simulink model "Bicopter_Dynamics"  (R2019a)
settings: Solver=ode4  StartTime=0.0  StopTime=5  FixedStep=0.0001  RelTol=1e-3
libraries: simulink x1
settings Model: Creator=crsmyth  LastModifiedBy=crs20

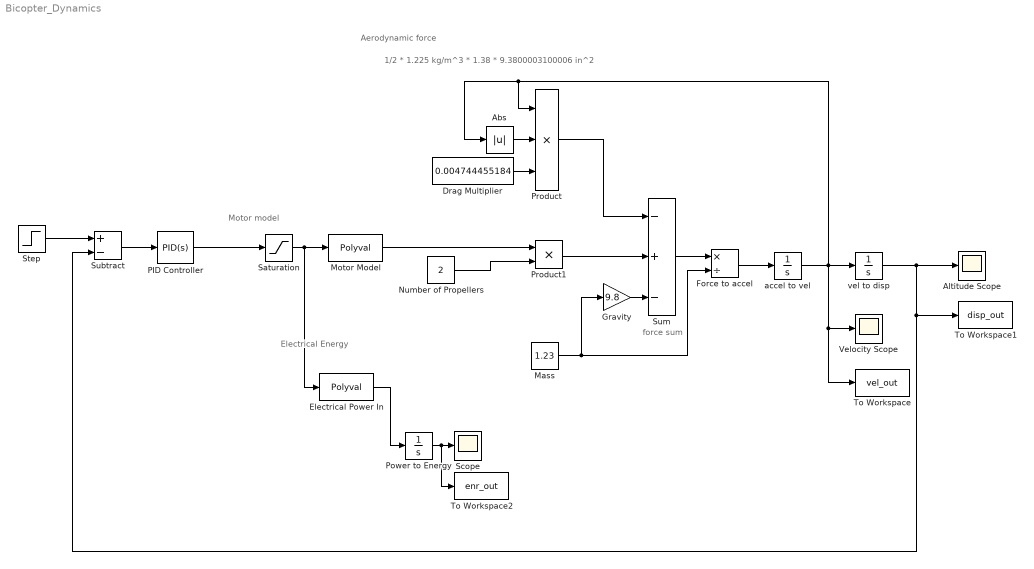
== system Bicopter_Dynamics ==
  note: Electrical Energy
  note: force sum
  note: Motor model
  note: Aerodynamic force
  note: 1/2 * 1.225 kg/m^3 * 1.38 * 9.3800003100006 in^2
  Abs : Abs
  Altitude Scope : Scope
  Drag Multiplier : Constant  Value=0.004744455184
  Electrical Power In : Polyval  Coefs=[2.956191832898671e+02, -6.235353126465623e+02, 3.330393150826374e+02]
  Force to accel : Product  Inputs=*/
  Gravity : Gain  Gain=9.8
  Mass : Constant  Value=1.23
  Motor Model : Polyval  Coefs=[4.843819998761814,-4.792311105872948,-0.068689974553541]
  Number of Propellers : Constant  Value=2
  PID Controller : simulink/Continuous/PID Controller  Controller=PID  Form=Parallel  TimeDomain=Continuous-time  SampleTime=-1  IntegratorMethod=Forward Euler  FilterMethod=Forward Euler  ControllerParametersSource=internal  P=1.5  I=1.3  D=0.3  UseFilter=on  N=10  TunerSelectOption=Transfer Function Based (PID Tuner App)  InitialConditionSource=internal  InitialConditionForIntegrator=0  InitialConditionForFilter=0  DifferentiatorICPrevScaledInput=0  ExternalReset=none  TrackingMode=off  Kt=1  LimitOutput=off  UpperSaturationLimit=inf  LowerSaturationLimit=-inf  LinearizeAsGain=on  AntiWindupMode=none  Kb=1  POutMin=[]  POutMax=[]  IOutMin=[]  IOutMax=[]  DOutMin=[]  DOutMax=[]  NOutMin=[]  NOutMax=[]  SumOutMin=[]  SumOutMax=[]  SaturationOutMin=[]  SaturationOutMax=[]  PParamMin=[]  PParamMax=[]  IParamMin=[]  IParamMax=[]  DParamMin=[]  DParamMax=[]  NParamMin=[]  NParamMax=[]  KbParamMin=[]  KbParamMax=[]  KtParamMin=[]  KtParamMax=[]  KbOutMin=[]  KbOutMax=[]  KtOutMin=[]  KtOutMax=[]  IntegratorOutMin=[]  IntegratorOutMax=[]  FilterOutMin=[]  FilterOutMax=[]  SumI1OutMin=[]  SumI1OutMax=[]  SumI2OutMin=[]  SumI2OutMax=[]  SumI3OutMin=[]  SumI3OutMax=[]  SumI4OutMin=[]  SumI4OutMax=[]  SumDOutMin=[]  SumDOutMax=[]  DifferentiatorOutMin=[]  DifferentiatorOutMax=[]  FilterDiffOutCoefMin=[]  FilterDiffOutCoefMax=[]  ReciprocalOutMin=[]  ReciprocalOutMax=[]  SumDenOutMin=[]  SumDenOutMax=[]  SumNumOutMin=[]  SumNumOutMax=[]  DivideOutMin=[]  DivideOutMax=[]  IntegratorContinuousStateAttributes=''  IntegratorStateMustResolveToSignalObject=off  IntegratorRTWStateStorageClass=Auto  FilterContinuousStateAttributes=''  FilterStateMustResolveToSignalObject=off  FilterRTWStateStorageClass=Auto  ParallelPVariant=InternalParameters  IdealPVariant=Disabled  IVariant=InternalParameters  DVariant=InternalParameters  IntegratorVariant=Continuous  SatVariant=Disabled  AWVariant=Passthrough  PCopyVariant=Disabled  TRVariant=Disabled  FdbkBlocksVariant=Forward  IdealPFdbkVariant=Disabled  SatFdbkVariant=Disabled  DerivativeFilterVariant=ContFilter  NVariant=InternalParameters  NCopyVariant=Disabled  FilterICVariant=InternalICsFilter  IntegratorICVariant=InternalICs  ExternalResetVariant=Disabled  TRSumVariant=Passthrough  SumFdbkVariant=Disabled  SumVariant=Sum_PID
  Power to Energy : Integrator
  Product : Product  Inputs=3
  Product1 : Product
  Saturation : Saturate  UpperLimit=2  LowerLimit=0
  Scope : Scope
  Step : Step  Time=0  After=2  SampleTime=0
  Subtract : Sum  Inputs=+-
  Sum : Sum  Inputs=-+-
  To Workspace : ToWorkspace  VariableName=vel_out  SampleTime=-1
      settings: Save2DSignal=2-D array (concatenate along first dimension)
  To Workspace1 : ToWorkspace  VariableName=disp_out  SampleTime=-1
      settings: Save2DSignal=2-D array (concatenate along first dimension)
  To Workspace2 : ToWorkspace  VariableName=enr_out  SaveFormat=Timeseries  SampleTime=-1
  Velocity Scope : Scope
  accel to vel : Integrator
  vel to disp : Integrator
  wires:
  Sum/1 -> Force to accel/1
  Mass/1 -> Gravity/1, Force to accel/2
  Force to accel/1 -> accel to vel/1
  Gravity/1 -> Sum/3
  Product/1 -> Sum/1
  Drag Multiplier/1 -> Product/3
  Abs/1 -> Product/2
  Product1/1 -> Sum/2
  Number of Propellers/1 -> Product1/2
  Motor Model/1 -> Product1/1
  accel to vel/1 -> vel to disp/1, Abs/1, Product/1, To Workspace/1, Velocity Scope/1
  vel to disp/1 -> To Workspace1/1, Subtract/2, Altitude Scope/1
  Electrical Power In/1 -> Power to Energy/1
  Power to Energy/1 -> To Workspace2/1, Scope/1
  Saturation/1 -> Electrical Power In/1, Motor Model/1
  PID Controller/1 -> Saturation/1
  Subtract/1 -> PID Controller/1
  Step/1 -> Subtract/1
